simulink library "Sim_Library"  (R2015b)
settings: Solver=ode45  SolverMode=SingleTasking  StartTime=0.0  StopTime=10.0  RelTol=1e-3
undefined symbols (not defined in the file): agent, CTRL, FRAME, k, k_throttle, l, ROTOR
libraries: Sim_Library x17, vrlib x2, aerolibutil x1
(part 2 of 2)

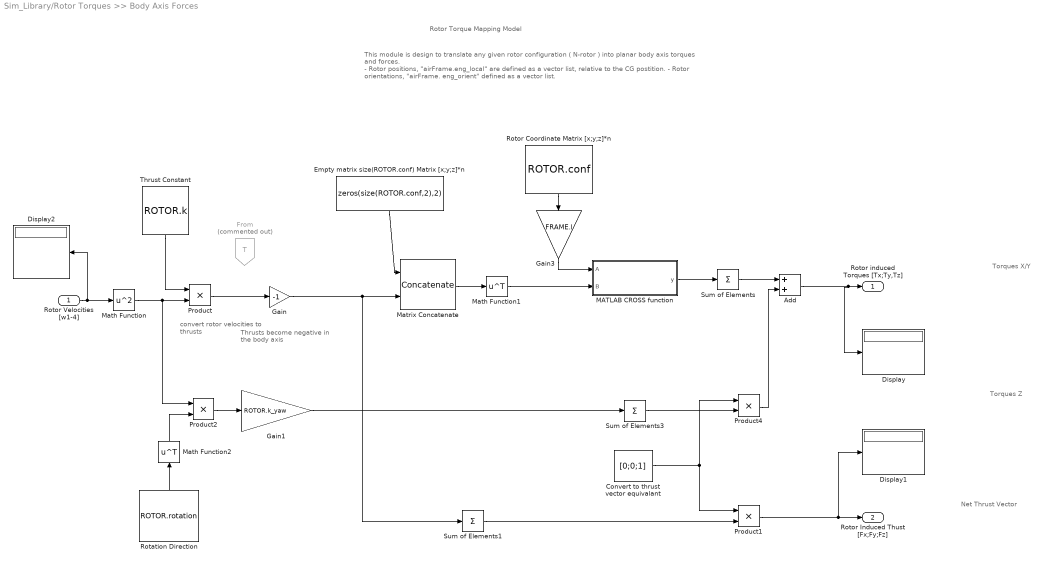
== system Sim_Library/Rotor Torques >> Body Axis Forces ==
  note: - Rotor positions, "airFrame.eng_local" are defined as a vector list, relative to the CG postition.
      | - Rotor orientations, "airFrame. eng_orient" defined as a vector list.
  note: This module is design to translate any given rotor configuration ( N-rotor ) into planar body axis torques and forces.
  note: Net Thrust Vector
  note: Torques Z
  note: Torques X/Y
  note: Thrusts become negative in the body axis
  note: Rotor Torque Mapping Model
  note: convert rotor velocities
      | to thrusts
  Rotor Velocities [w1-4] : Inport
  Add : Sum
  Convert to thrust vector equivalant : Constant  Value=[0;0;1]  VectorParams1D=off
  Display : Display
  Display1 : Display
  Display2 : Display
  Empty matrix size(ROTOR.conf) Matrix [x;y;z]*n : Constant  Value=zeros(size(ROTOR.conf,2),2)  VectorParams1D=off
  From : From  Commented=on  GotoTag=T  TagVisibility=global
  Gain : Gain  Gain=-1
  Gain1 : Gain  Gain=ROTOR.k_yaw
  Gain3 : Gain  Gain=FRAME.l
  MATLAB CROSS function : MATLAB Function  TreatAsAtomicUnit=on
  Math Function : Math  Operator=square  SaturateOnIntegerOverflow=on
  Math Function1 : Math  Operator=transpose  SaturateOnIntegerOverflow=on
  Math Function2 : Math  Operator=transpose  SaturateOnIntegerOverflow=on
  Matrix Concatenate : Concatenate  Mode=Multidimensional array  ConcatenateDimension=2
  Product{,1..2,4} (4 alike) : Product
  Rotation Direction : Constant  Value=ROTOR.rotation  VectorParams1D=off
  Rotor Coordinate Matrix [x;y;z]*n : Constant  Value=ROTOR.conf  VectorParams1D=off
  Sum of Elements : Sum  Inputs=+  CollapseMode=Specified dimension  CollapseDim=2
  Sum of Elements1 : Sum  Inputs=+  CollapseMode=Specified dimension
  Sum of Elements3 : Sum  Inputs=+  CollapseMode=Specified dimension
  Thrust Constant : Constant  Value=ROTOR.k  VectorParams1D=off
  Rotor induced Torques [Tx;Ty,Tz] : Outport
  Rotor Induced Thust [Fx;Fy;Fz] : Outport  Port=2
  wires:
  Product/1 -> Gain/1
  Product2/1 -> Gain1/1
  Add/1 -> Rotor induced Torques [Tx;Ty,Tz]/1, Display/1
  Product1/1 -> Rotor Induced Thust [Fx;Fy;Fz]/1, Display1/1
  Product4/1 -> Add/2
  Sum of Elements3/1 -> Product4/2
  Rotor Coordinate Matrix [x;y;z]*n/1 -> Gain3/1
  Gain3/1 -> MATLAB CROSS function/1(A)
  Gain1/1 -> Sum of Elements3/1
  Math Function2/1 -> Product2/2
  Rotation Direction/1 -> Math Function2/1
  Thrust Constant/1 -> Product/1
  Sum of Elements1/1 -> Product1/2
  Convert to thrust vector equivalant/1 -> Product4/1, Product1/1
  Sum of Elements/1 -> Add/1
  Gain/1 -> Matrix Concatenate/2, Sum of Elements1/1
  MATLAB CROSS function/1(y) -> Sum of Elements/1
  Math Function1/1 -> MATLAB CROSS function/2(B)
  Matrix Concatenate/1 -> Math Function1/1
  Empty matrix size(ROTOR.conf) Matrix [x;y;z]*n/1 -> Matrix Concatenate/1
  Math Function/1 -> Product2/1, Product/2
  Rotor Velocities [w1-4]/1 -> Display2/1, Math Function/1

== system Sim_Library/Simple Altitude PID ==
  note: Altitude Hold Controller
  note: Output U0; Height
      | adjustment control signal
  Target Height [h] m : Inport
  Meausured Height [h] m : Inport  Port=2
  Altitude Integrator : Integrator
  Altitude Differencial Gain : Gain  Gain=agent.altitude_kd
  Altitude Integral Gain : Gain  Gain=agent.altitude_ki
  Altitude Proportional Gain : Gain  Gain=agent.altitude_kp
  Derivative : Derivative
  Display : Display
  Scope : Scope
  Subtract : Sum  Inputs=-+
  Sum1 : Sum  Inputs=+++
  Alttitude Correction [T] N : Outport
  wires:
  Derivative/1 -> Sum1/3
  Altitude Differencial Gain/1 -> Derivative/1
  Subtract/1 -> Altitude Integral Gain/1, Altitude Proportional Gain/1, Altitude Differencial Gain/1
  Altitude Integrator/1 -> Sum1/2
  Altitude Integral Gain/1 -> Altitude Integrator/1
  Target Height [h] m/1 -> Subtract/2
  Meausured Height [h] m/1 -> Subtract/1
  Sum1/1 -> Alttitude Correction [T] N/1, Scope/1, Display/1
  Altitude Proportional Gain/1 -> Sum1/1

== system Sim_Library/Temperature Relation ==
  note: Atmospheric Temperature Relationship
  note: Stratospheric Relations
  note: Trophosphere Relations
  Altitude [m] : Inport
  Divide : Product  Inputs=*/
  Lapse Rate1 : Gain  Gain=0.0065
  Sea Level Temperature [K] : Constant  Value=288.15
  Switch : Switch  Criteria=u2 > Threshold  Threshold=11000
  T0--lam*h* : Sum  Inputs=-+
  Tropo-pause [m] : Constant  Value=11000
  Temperature [K] : Outport
  Relative Temperature : Outport  Port=2
  wires:
  T0--lam*h*/1 -> Temperature [K]/1, Divide/1
  Switch/1 -> Lapse Rate1/1
  Tropo-pause [m]/1 -> Switch/1
  Altitude [m]/1 -> Switch/2, Switch/3
  Lapse Rate1/1 -> T0--lam*h*/1
  Sea Level Temperature [K]/1 -> Divide/2, T0--lam*h*/2
  Divide/1 -> Relative Temperature/1

== system Sim_Library/2 Tier PID Attitude + Rate Controller/3D Rate Controller Layer ==
  note: 3D PID Rate Controller
  Measured Rates [si;th;pi] dot : Inport
  Target Rates [si;th;pi] dot : Inport  Port=2
  " " : Product  Multiplication=Matrix(*)
  1 : Product  Multiplication=Matrix(*)
  D Gains [si,th,pi] : Product  Multiplication=Matrix(*)
  Derivative Gains : FromWorkspace  VariableName=[Dsi,Dth,Dph]  SampleTime=0
  Error [si,th,pi] : Sum  Inputs=-+
  I Gains [si,th,pi] : Product  Multiplication=Matrix(*)
  Integral Gains : FromWorkspace  VariableName=[Psi,Pth,Pph]  SampleTime=0
  Integrator : Integrator
  P Gains [si,th,pi] : Product  Multiplication=Matrix(*)
  Proportional Gains : FromWorkspace  VariableName=[Psi,Pth,Pph]  SampleTime=0
  Setpoint Gains (Derivative) : FromWorkspace  VariableName=[1;1;1]  SampleTime=0
  Setpoint Gains (Proportional) : FromWorkspace  VariableName=[1;1;1]  SampleTime=0
  Sum : Sum  Inputs=+-
  Sum1 : Sum  Inputs=-+
  Sum2 : Sum  Inputs=+++
  PID Outputs [Ksi;Kth;Kpi] : Outport
  wires:
  1/1 -> Sum1/2
  I Gains [si,th,pi]/1 -> Integrator/1
  Proportional Gains/1 -> P Gains [si,th,pi]/1
  Error [si,th,pi]/1 -> I Gains [si,th,pi]/2
  Integral Gains/1 -> I Gains [si,th,pi]/1
  Sum1/1 -> D Gains [si,th,pi]/1
  Integrator/1 -> Sum2/2
  Setpoint Gains (Derivative)/1 -> 1/2
  " "/1 -> Sum/1
  Setpoint Gains (Proportional)/1 -> " "/1
  Derivative Gains/1 -> D Gains [si,th,pi]/2
  Sum2/1 -> PID Outputs [Ksi;Kth;Kpi]/1
  P Gains [si,th,pi]/1 -> Sum2/1
  D Gains [si,th,pi]/1 -> Sum2/3
  Measured Rates [si;th;pi] dot/1 -> Error [si,th,pi]/1, Sum/2, Sum1/1, " "/2, 1/1
  Target Rates [si;th;pi] dot/1 -> Error [si,th,pi]/2
  Sum/1 -> P Gains [si,th,pi]/2

== matlab function Sim_Library/Navigational PID/MATLAB Inverse ==
  data: u input; y output
function y = fcn(u)
%#codegen

y = u^-1;

== matlab function Sim_Library/Rotor Torques >> Body Axis Forces/MATLAB CROSS function ==
  data: A input; y output; B input
function y = MAT_crossproduct(A,B)
%#Calculate the matlab cross product 
y = cross(A,B,1);
